simulink model "Simulink_Model_Q2"  (R2015a)
settings: Solver=ode45  StartTime=0.0  StopTime=45  MaxStep=0.01  RelTol=1e-3
values from neighbouring files (symbols this model uses):
  A = 2.2    [PBA1_script.m]    (also in PBA3_1.m = simplify(subs(jacobian(F_x, x), x_T, equ)); cruise_control.m; gyro_pendulum.m = simplify(subs(jacobian(F_x, x), x_T, equ)); helicopter_eom.m = [A11, A12; A21])
  alpha = {40, 35, 16, 12, 10}    [PBA1_script.m]    (also in cruise_control.m)
  beta = 0.35    [PBA1_script.m]    (also in cruise_control.m)
  Cd = 0.36    [PBA1_script.m]    (also in cruise_control.m)
  Cr = 0.01    [PBA1_script.m]    (also in cruise_control.m)
  g = 9.81    [Bicycle_whipple.m]    (also in PBA1_script.m; PBA3_2_script.m; PBA3_4_script.m; cruise_control.m)
  m = 1200    [PBA1_script.m]    (also in PBA3_2_script.m = 80; PBA3_4_script.m = 80; cruise_control.m = 1000)
  p = 1.3    [PBA1_script.m]    (also in cruise_control.m; massandcart.m = 0)
  Tm = 200    [PBA1_script.m]    (also in cruise_control.m)
  wm = 450    [cruise_control.m]
libraries: simulink_extras x1
settings Model: Creator=Callum  LastModifiedBy=Owner
settings HardwareCC: TargetLongLongMode=on  TargetIntDivRoundTo=Zero  TargetEndianess=LittleEndian  TargetHWDeviceType=MATLAB Host  ProdEqTarget=off
settings RTWCC: SystemTargetFile=rsim.tlc  TemplateMakefile=rsim_default_tmf  Description=Rapid Simulation Target
settings RSimTargetCC: ERTMultiwordTypeDef=System defined  ERTMultiwordLength=256

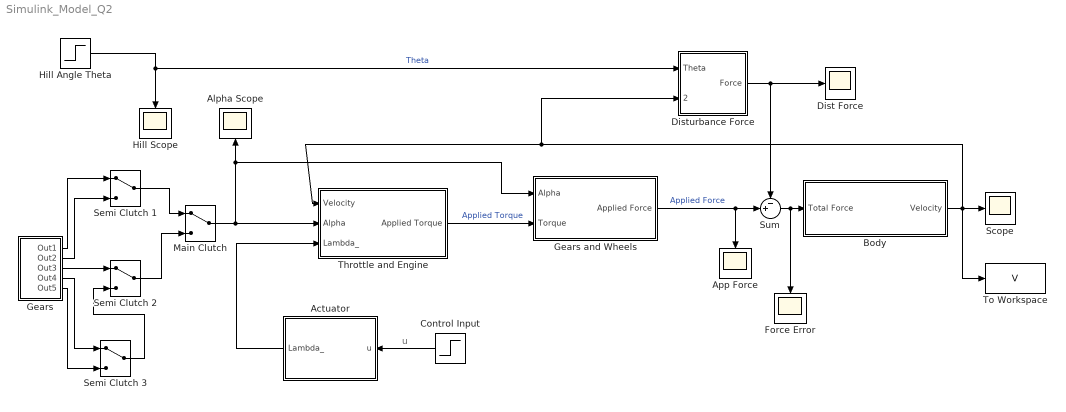
== system Simulink_Model_Q2 ==
  note: u
  Actuator : Subsystem
  Alpha Scope : Scope
      settings: SaveName=ScopeData3
  App Force : Scope
      settings: SaveName=ScopeData7
  Body : Subsystem
  Control Input : Step  Time=5  After=0.5  SampleTime=0
  Dist Force : Scope
      settings: SaveName=ScopeData6
  Disturbance Force : Subsystem
  Force Error : Scope
      settings: SaveName=ScopeData8
  Gears : Subsystem
  Gears and Wheels : Subsystem
  Hill Scope : Scope
      settings: SaveName=ScopeData5
  Hill Angle Theta : Step  Time=0  After=0  SampleTime=0
  Main Clutch : ManualSwitch
  Scope : Scope
  Semi Clutch 1 : ManualSwitch
  Semi Clutch 2 : ManualSwitch
  Semi Clutch 3 : ManualSwitch
  Sum : Sum  Inputs=-+|
  Throttle and Engine : Subsystem
  To Workspace : ToWorkspace  VariableName=V  SaveFormat=Timeseries  SampleTime=-1
  wires:
  Hill Angle Theta/1 -> Hill Scope/1, Disturbance Force/1(Theta)  "Theta"
  Disturbance Force/1(Force) -> Dist Force/1, Sum/1
  Actuator/1(Lambda_) -> Throttle and Engine/3(Lambda_)
  Body/1(Velocity) -> Scope/1, To Workspace/1, Disturbance Force/2(Velocity), Throttle and Engine/1(Velocity)
  Sum/1 -> Body/1(Total Force), Force Error/1
  Throttle and Engine/1(Applied Torque) -> Gears and Wheels/2(Torque)  "Applied Torque"
  Gears and Wheels/1(Applied Force) -> Sum/2, App Force/1  "Applied Force"
  Semi Clutch 1/1 -> Main Clutch/1
  Semi Clutch 2/1 -> Main Clutch/2
  Semi Clutch 3/1 -> Semi Clutch 2/2
  Main Clutch/1 -> Gears and Wheels/1(Alpha), Alpha Scope/1, Throttle and Engine/2(Alpha)
  Gears/1(Out1) -> Semi Clutch 1/1
  Gears/2(Out2) -> Semi Clutch 1/2
  Gears/3(Out3) -> Semi Clutch 2/1
  Gears/4(Out4) -> Semi Clutch 3/1
  Gears/5(Out5) -> Semi Clutch 3/2
  Control Input/1 -> Actuator/1(u)

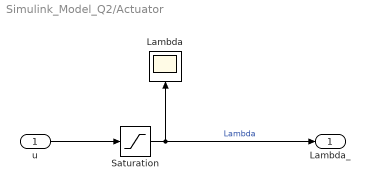
== system Simulink_Model_Q2/Actuator ==
  u : Inport
  Lambda : Scope
      settings: SaveName=ScopeData4
  Saturation : Saturate  UpperLimit=1  LowerLimit=0
  Lambda_ : Outport
  wires:
  Saturation/1 -> Lambda_/1, Lambda/1  "Lambda"
  u/1 -> Saturation/1

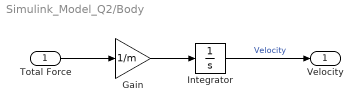
== system Simulink_Model_Q2/Body ==
  Total Force : Inport
  Gain : Gain  Gain=1/m
  Integrator : Integrator
  Velocity : Outport
  wires:
  Total Force/1 -> Gain/1
  Gain/1 -> Integrator/1
  Integrator/1 -> Velocity/1  "Velocity"

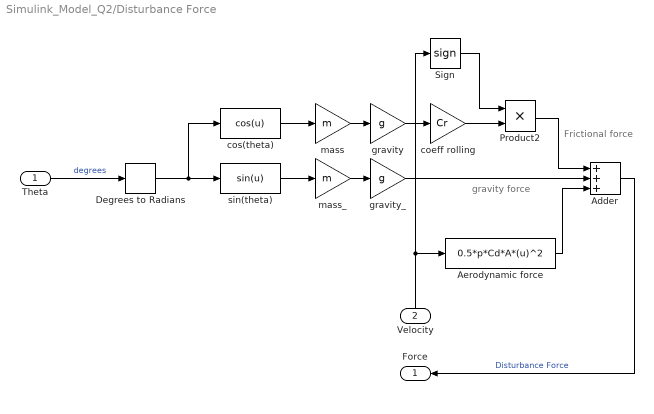
== system Simulink_Model_Q2/Disturbance Force ==
  note: Frictional force
  note: gravity force
  Theta : Inport
  Velocity : Inport  Port=2
  Adder : Sum  Inputs=+++
  Aerodynamic force : Fcn  Expr=0.5*p*Cd*A*(u)^2
  Degrees to Radians : simulink_extras/Transformations/Degrees to Radians
  Product2 : Product
  Sign : Signum
  coeff rolling : Gain  Gain=Cr
  cos(theta) : Fcn  Expr=cos(u)
  gravity : Gain  Gain=g
  gravity_ : Gain  Gain=g
  mass : Gain  Gain=m
  mass_ : Gain  Gain=m
  sin(theta) : Fcn  Expr=sin(u)
  Force : Outport
  wires:
  Adder/1 -> Force/1  "Disturbance Force"
  Sign/1 -> Product2/1
  gravity/1 -> coeff rolling/1
  mass/1 -> gravity/1
  Aerodynamic force/1 -> Adder/3
  Product2/1 -> Adder/1
  mass_/1 -> gravity_/1
  gravity_/1 -> Adder/2
  coeff rolling/1 -> Product2/2
  cos(theta)/1 -> mass/1
  sin(theta)/1 -> mass_/1
  Degrees to Radians/1 -> sin(theta)/1, cos(theta)/1
  Velocity/1 -> Sign/1, Aerodynamic force/1
  Theta/1 -> Degrees to Radians/1  "degrees"

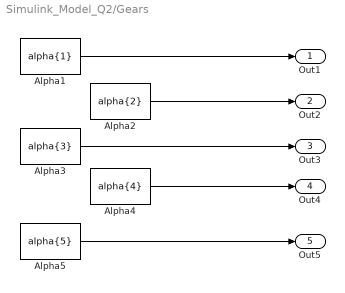
== system Simulink_Model_Q2/Gears ==
  Alpha1 : Constant  Value=alpha{1}
  Alpha2 : Constant  Value=alpha{2}
  Alpha3 : Constant  Value=alpha{3}
  Alpha4 : Constant  Value=alpha{4}
  Alpha5 : Constant  Value=alpha{5}
  Out1 : Outport
  Out2 : Outport  Port=2
  Out3 : Outport  Port=3
  Out4 : Outport  Port=4
  Out5 : Outport  Port=5
  wires:
  Alpha5/1 -> Out5/1
  Alpha4/1 -> Out4/1
  Alpha2/1 -> Out2/1
  Alpha1/1 -> Out1/1
  Alpha3/1 -> Out3/1

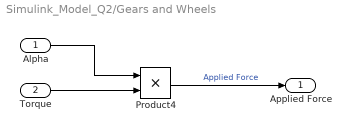
== system Simulink_Model_Q2/Gears and Wheels ==
  Alpha : Inport
  Torque : Inport  Port=2
  Product4 : Product
  Applied Force : Outport
  wires:
  Product4/1 -> Applied Force/1  "Applied Force"
  Torque/1 -> Product4/2
  Alpha/1 -> Product4/1

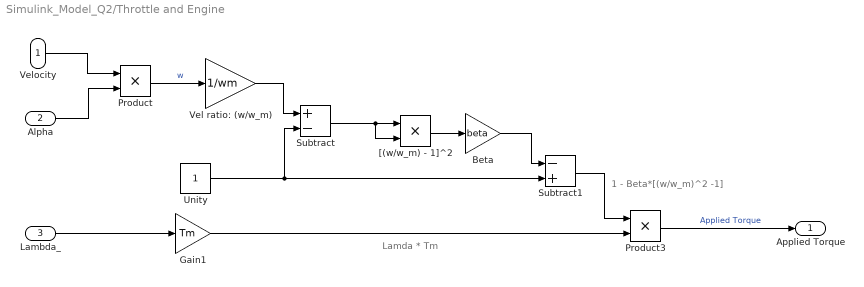
== system Simulink_Model_Q2/Throttle and Engine ==
  note: 1 - Beta*[(w/w_m)^2 -1]
  note: Lamda * Tm
  Velocity : Inport
  Alpha : Inport  Port=2
  Lambda_ : Inport  Port=3
  Beta : Gain  Gain=beta
  Gain1 : Gain  Gain=Tm
  Product : Product
  Product3 : Product
  Subtract : Sum  Inputs=+-
  Subtract1 : Sum  Inputs=-+
  Unity : Constant
  Vel ratio: (w/w_m) : Gain  Gain=1/wm
  "[(w/w_m) - 1]^2" : Product
  Applied Torque : Outport
  wires:
  Product/1 -> Vel ratio: (w/w_m)/1  "w"
  Vel ratio: (w/w_m)/1 -> Subtract/1
  Unity/1 -> Subtract/2, Subtract1/2
  Subtract/1 -> "[(w/w_m) - 1]^2"/2, "[(w/w_m) - 1]^2"/1
  "[(w/w_m) - 1]^2"/1 -> Beta/1
  Beta/1 -> Subtract1/1
  Subtract1/1 -> Product3/1
  Product3/1 -> Applied Torque/1  "Applied Torque"
  Gain1/1 -> Product3/2
  Alpha/1 -> Product/2
  Velocity/1 -> Product/1
  Lambda_/1 -> Gain1/1
